simulink model "bio_matfunc_on_time_calc"  (R2017b)
settings: Solver=VariableStepAuto  StartTime=0.0  StopTime=10.0  RelTol=1e-3
settings Model: Creator=ktrinh  LastModifiedBy=ktrinh

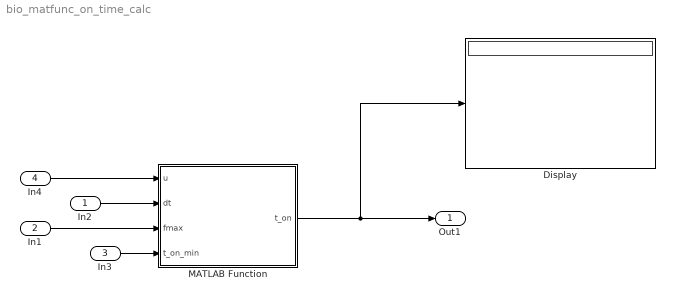
== system bio_matfunc_on_time_calc ==
  In2 : Inport  OutDataTypeStr=double  PortDimensions=1
  In1 : Inport  Port=2  OutDataTypeStr=double  PortDimensions=1
  In3 : Inport  Port=3  OutDataTypeStr=double  PortDimensions=1
  In4 : Inport  Port=4  OutDataTypeStr=double  PortDimensions=6
  Display : Display
  MATLAB Function : MATLAB Function  TreatAsAtomicUnit=on
  Out1 : Outport
  wires:
  In2/1 -> MATLAB Function/2(dt)
  In1/1 -> MATLAB Function/3(fmax)
  In3/1 -> MATLAB Function/4(t_on_min)
  In4/1 -> MATLAB Function/1(u)
  MATLAB Function/1(t_on) -> Display/1, Out1/1

== matlab function bio_matfunc_on_time_calc/MATLAB Function ==
  data: u input; t_on output; dt input; fmax input; t_on_min input
function t_on = on_time_calc(u,dt,fmax,t_on_min)
%#codegen

t_on = zeros(6,1);
for i = 1:6
    t_on(i) = u(i)*dt/fmax;
    if t_on(i) < t_on_min
        t_on(i) = 0;
    elseif t_on(i) > dt
        t_on(i) = dt;
    end
end
